simulink model "sine"  (R2022b)
settings: Solver=VariableStepAuto  StartTime=0.0  StopTime=10.0  RelTol=1e-3
settings Model: Creator=OXYGEN  LastModifiedBy=OXYGEN

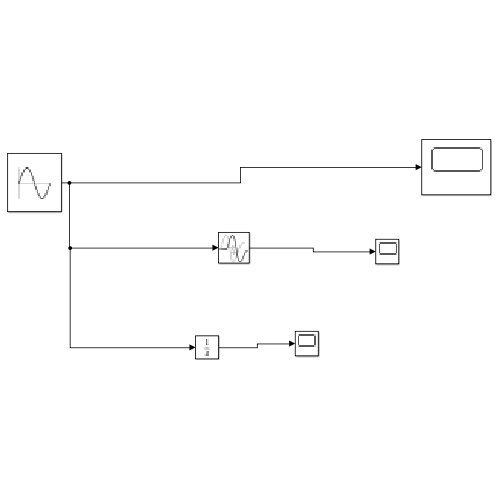
[thumbnail: Simulink's stored preview of the top-level diagram]
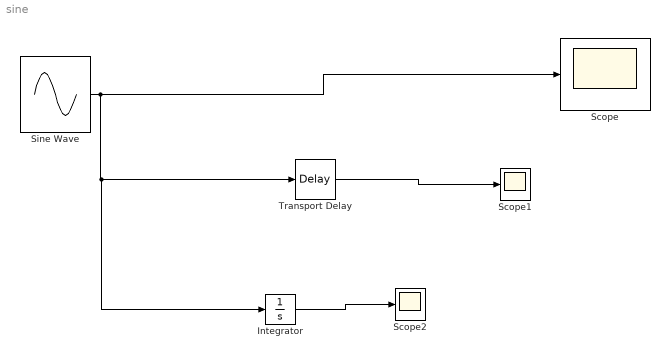
== system sine ==
  Integrator : Integrator
  Scope : Scope
  Scope1 : Scope
  Scope2 : Scope
  Sine Wave : Sin  SampleTime=0
  Transport Delay : TransportDelay
  wires:
  Sine Wave/1 -> Integrator/1, Transport Delay/1, Scope/1
  Transport Delay/1 -> Scope1/1
  Integrator/1 -> Scope2/1
